simulink model "soccerbot"  (R2017b)
settings: Solver=FixedStepDiscrete  StartTime=0.0  StopTime=10  FixedStep=0.01  RelTol=1e-3
PreLoadFcn:
  | clear;
  | 
  | % Sample times
  | sampleTime = 0.2;
  | 
  | % Control parameters
  | ctrlParam1 = 2;
  | ctrlParam2 = 3.5;
  | 
  | loadIpAddresses;
InitFcn:
  | loadFixedTrajectories;
model workspace (MAT data in the model file):
  SL_ROS_VariableLengthArrays_MaxSizes : struct (value not decoded)
  ctrlParam1 = 1
  ctrlParam2 = 1.5
  sampleTime = 0.01
values from neighbouring files (symbols this model uses):
  findBallTraj = zeros(1000,20)    [loadFixedTrajectories.m]
  getUpBackTraj = getUpBackTraj'    [loadFixedTrajectories.m]
  getUpFrontTraj = getUpFrontTraj'    [loadFixedTrajectories.m]    (also in loadModelData.m)
  motorCalibration = [0;0;0;0;0;0;0;0;0;0;0;0;0;0;0;0;0;0;0;0]    [loadFixedTrajectories.m]    (also in loadRobot.m; soccer_strategy_setup.m)
  prepareToWalkTraj = spline(t, prepareToWalkWayPoints, prepareToWalkTrajTime)'    [loadFixedTrajectories.m]
undefined symbols (not defined in the file or in its folder): customState, DiscIntNeverNeededParam, resting, walkTraj
libraries: simulink x102, robotlib x5, sharedtransform x1, visionsinks x1
(part 2 of 2)

== stateflow chart soccerbot/Robot Decision ==
  state StatusOk
    state Ready
      entry: trajAction = 1
    state LookForBall
      entry: trajAction = 5; trigger = 0;
    state PrepareToWalk
      entry: trajAction = 6;
    state Walking
      entry: trajAction = 0; trigger = 1;
      wayPoints = findWayPoints(currentPose, obstacles, destinationPose);
    (default) -> Ready
    Ready -> LookForBall : [after(3,sec)]
    LookForBall -> LookForBall [order 1] : [ballFound==0 && after(10,sec)]
    Walking -> LookForBall : [status == 1]
    LookForBall -> PrepareToWalk [order 2] : [ballFound == 1 && after(1,sec)]
    PrepareToWalk -> Walking : [status == 1]
  state FallenFront
    entry: trajAction = 3;
  state FallenBack
    entry: trajAction = 4;
  FallenFront -> StatusOk [order 1] : [status == 1 && fallenBack ~= 1 && fallenFront ~= 1]
  (default) -> StatusOk
  FallenFront -> FallenFront [order 3] : [status == 1 && fallenFront == 1]
  StatusOk -> FallenFront [order 2] : [fallenFront == 1]
  FallenFront -> FallenBack [order 2] : [status == 1 && fallenBack == 1]
  FallenBack -> FallenFront [order 2] : [status == 1 && fallenFront == 1]
  StatusOk -> FallenBack [order 1] : [fallenBack == 1]
  FallenBack -> FallenBack [order 1] : [status == 1 && fallenBack== 1]
  data: curPose function_input; obs function_input; destPos function_input; waypoints function_output; fallenBack input; fallenFront input; ballFound input; currentPose input; destinationPose input; obstacles input; status input; trajAction output; wayPoints output; trigger output
  function waypoints = findWayPoints(curPose, obs, destPos):
    | function waypoints = findWayPoints(curPose, obs, destPos)
    |     
    |     % Hardcoded poses
    |     pose2 = [0.1, 0, 0, 0, 0.04];
    |     pose3 = [0.4, 0.2, 0, 0, 0.04];
    |     pose4 = [0.4, -0.2, 0, -pi, 0.04];
    |     pose5 = [0.1, 0, 0, -pi, 0.04];
    |     pose6 = [0, 0, 0, -pi, 0.0];
    |     
    |     waypoints = [pose2, pose3, pose4, pose5, pose6];
    | end
